simulink model "TRAS_nonlinear_controller"  (R2013a)
settings: Solver=ode5  SolverMode=SingleTasking  StartTime=0.0  StopTime=stop_time  FixedStep=sampling_time  RelTol=1e-3  AbsTol=1e-6
values from neighbouring files (symbols this model uses):
  A = 0.0552    [momentsOfInertia.m]
  B = 0.0599    [momentsOfInertia.m]
  C = 0.0084    [momentsOfInertia.m]
  D = (mmr + mms + mm / 3) * lm^2 + (mtr + mts + mt / 3) * lt^2    (= 0.0224143186667)    [momentsOfInertia.m]
  derivative_pole_tc = 10 * sampling_time    (= 0.1)    [TRAS_closed_loop.m]
  F = mms * rms^2 + mts * rts^2    (= 0.002355075)    [momentsOfInertia.m]
  Fh_force_grid = polyval(Fh, Fh_omega_grid)    [thrustForcesDependencies.m]
  Fh_omega_grid = linspace(-8000, 8000, 1e4)    [thrustForcesDependencies.m]
  Fv_force_grid = polyval(Fv, Fv_omega_grid)    [thrustForcesDependencies.m]
  Fv_omega_grid = linspace(-4000, 4000, 1e4)    [thrustForcesDependencies.m]
  g = 9.81    [TRAS_closed_loop.m]    (also in TRAS_controller.m; TRAS_process.m)
  Jv = D + E + F    (= 0.0253918936667)    [momentsOfInertia.m]
  kdh = 2 * zetah * wnh + poleh    (= 5.07276507277)    [TRAS_closed_loop.m]
  kdv = 2 * zetav * wnv + polev    (= 5.76397515528)    [TRAS_closed_loop.m]
  ki_inner = wn_inner^2    (= 19.7530864198)    [TRAS_closed_loop.m]
  kih = poleh * wnh^2    (= 2.0128563833)    [TRAS_closed_loop.m]
  kiv = polev * wnv^2    (= 3.43518684699)    [TRAS_closed_loop.m]
  kp_inner = 2 * zeta_inner * wn_inner    (= 8)    [TRAS_closed_loop.m]
  kph = wnh^2 + 2 * zetah * wnh * poleh    (= 6.9847554255)    [TRAS_closed_loop.m]
  kpv = wnv^2 + 2 * zetav * wnv * polev    (= 8.93792677752)    [TRAS_closed_loop.m]
  L = (mmr + mms + mm / 4) * lm^2 + (mtr + mts + mt / 4) * lt^2 - mcb * lcb^2 - mb / 4 * lb^2    (= 0.021593306)    [momentsOfInertia.m]
  lm = 0.202    [momentsOfInertia.m]
  lt = 0.216    [momentsOfInertia.m]
undefined symbols (not defined in the file): rtdac4pcibaseaddress
settings Model: SimulationMode=external  ExtModeTrigDuration=12000  ExtModeTrigLevel=0.400000  Creator=jims  LastModifiedBy=calc2
settings DataIOCC: ExternalInput=[]  InitialState=[]  LimitDataPoints=off  MaxDataPoints=5000  SignalLoggingSaveFormat=ModelDataLogs  SaveOutput=off  SaveTime=off  SignalLoggingName=sigsOut
settings OptimizationCC: BooleanDataType=off  ExpressionDepthLimit=2147483647  InitFltsAndDblsToZero=on
settings DebuggingCC: SaveWithParameterizedLinksMsg=none  MergeDetectMultiDrivingBlocksExec=error  SolverPrmCheckMsg=none  MultiTaskDSMMsg=warning  MultiTaskCondExecSysMsg=none  IntegerOverflowMsg=none  FcnCallInpInsideContextMsg=EnableAllAsWarning  StrictBusMsg=None
settings HardwareCC: TargetEndianess=LittleEndian  TargetHWDeviceType=MATLAB Host
settings RTWCC: SystemTargetFile=rtwin.tlc  TemplateMakefile=rtwin.tmf  Description=Real-Time Windows Target  ProcessScript=rtwin_make_rtw_hook  IncludeERTFirstTime=on
settings RTWinTargetCC: TargetFcnLib=ansi_tfl_tmw.mat  TargetLibSuffix=_rtwin.lib  TargetPreCompLibLocation=C:\Program Files\MATLAB\R2013a\toolbox\rtw\targets\rtwin\lib\win32  CodeReplacementLibrary=ANSI_C  ModelReferenceCompliant=off  CompOptLevelCompliant=off  RTWinDir=C:/PROGRA~1/MATLAB/R2013a/toolbox/rtw/targets/rtwin  TargetArch=win32

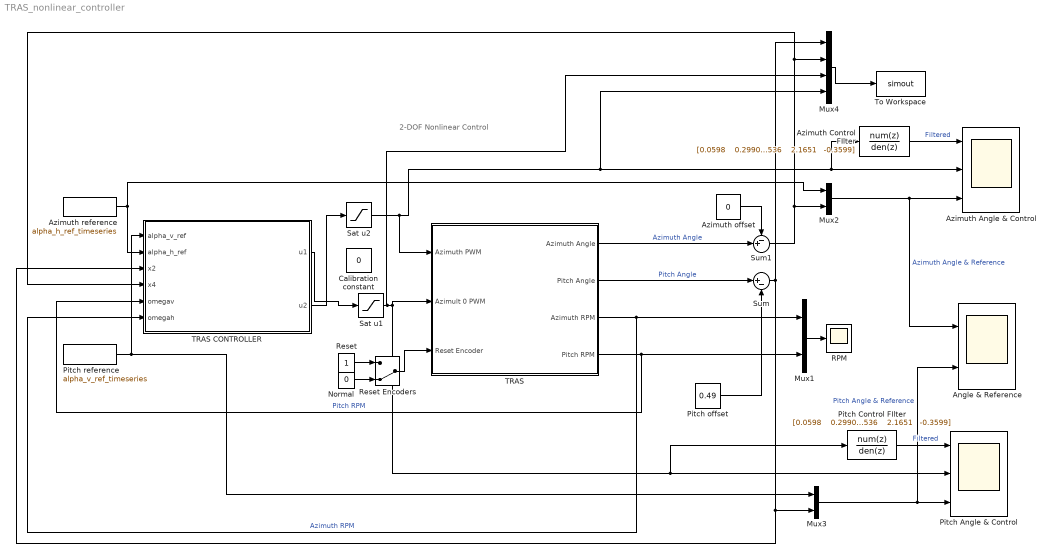
== system TRAS_nonlinear_controller ==
  note: 2-DOF Nonlinear Control
  Angle & Reference : Scope  NumInputPorts=2
      settings: TimeRange=60  YMin=-0.6~-0.55  YMax=0.8~0.55  SaveName=AngleReference_  MaxDataPoints=12000
  Azimuth Angle & Control : Scope  NumInputPorts=3
      settings: TimeRange=90  YMin=-0.4~-0.5~-1  YMax=-0.225~0.5~1  SaveName=AngleCtrl_  MaxDataPoints=12000
  Azimuth Control FIlter : DiscreteTransferFcn  Numerator="[0.0598    0.2990    0.5980    0.5980    0.2990    0.0598] * 1e-3"  Denominator="[1.0000   -3.9845    6.4349   -5.2536    2.1651   -0.3599]"  SampleTime=0.01
  Azimuth offset : Constant  Value=0
  "Azimuth reference " : FromWorkspace  VariableName=alpha_h_ref_timeseries  SampleTime=0
  Calibration constant : Constant  Value=0
  Mux1 : Mux  Inputs=2
  Mux2 : Mux  Inputs=2
  Mux3 : Mux  Inputs=2
  Mux4 : Mux
  Normal : Constant  Value=0
  Pitch Angle & Control : Scope  NumInputPorts=3
      settings: TimeRange=90  YMin=2.77556e-17~-0.1~-0.5  YMax=0.75~0.9~0.35  SaveName=AngleCtrl1_  MaxDataPoints=12000
  Pitch Control FIlter : DiscreteTransferFcn  Numerator="[0.0598    0.2990    0.5980    0.5980    0.2990    0.0598] * 1e-3"  Denominator="[1.0000   -3.9845    6.4349   -5.2536    2.1651   -0.3599]"  SampleTime=0.01
  Pitch offset : Constant  Value=0.49
  Pitch reference : FromWorkspace  VariableName=alpha_v_ref_timeseries  SampleTime=0
  RPM : Scope
      settings: TimeRange=90  YMin=-6000  YMax=7000  SaveName=RPM_  MaxDataPoints=12000
  Reset : Constant
  Reset Encoders : ManualSwitch  CurrentSetting=0
  Sat u1 : Saturate  UpperLimit=1  LowerLimit=-1
  Sat u2 : Saturate  UpperLimit=1  LowerLimit=-1
  Sum : Sum  Inputs=|+-
  Sum1 : Sum  Inputs=-+|
  TRAS : Subsystem  mask{BaseAddress=rtdac4pcibaseaddress, T0=0.01}
      mask prompts: BaseAddress "Base Address:"; T0 "Sampling Period:"
      mask Display: image(imread('TRAS.JPG'))
  TRAS CONTROLLER : Subsystem
  To Workspace : ToWorkspace  VariableName=simout  SampleTime=-1  SaveFormat=Structure With Time
  wires:
  Pitch Control FIlter/1 -> Pitch Angle & Control/1  "Filtered"
  Mux3/1 -> Pitch Angle & Control/3, Angle & Reference/2  "Pitch Angle & Reference"
  Mux1/1 -> RPM/1
  Sat u2/1 -> TRAS/1(Azimuth PWM), Mux4/4, Azimuth Angle & Control/2, Azimuth Control FIlter/1
  Sat u1/1 -> Mux4/3, TRAS/2(Azimult 0 PWM), Pitch Angle & Control/2, Pitch Control FIlter/1
  Azimuth Control FIlter/1 -> Azimuth Angle & Control/1  "Filtered"
  Mux2/1 -> Azimuth Angle & Control/3, Angle & Reference/1  "Azimuth Angle & Reference"
  Reset Encoders/1 -> TRAS/3(Reset Encoder)
  Reset/1 -> Reset Encoders/1
  Normal/1 -> Reset Encoders/2
  TRAS/4(Pitch RPM) -> TRAS CONTROLLER/5(omegav), Mux1/2  "Pitch RPM"
  TRAS/3(Azimuth RPM) -> TRAS CONTROLLER/6(omegah), Mux1/1  "Azimuth RPM"
  "Azimuth reference "/1 -> TRAS CONTROLLER/2(alpha_h_ref), Mux2/1
  Pitch reference/1 -> TRAS CONTROLLER/1(alpha_v_ref), Mux3/1
  Sum/1 -> TRAS CONTROLLER/3(x2), Mux3/2, Mux4/1
  Pitch offset/1 -> Sum/2
  Mux4/1 -> To Workspace/1
  Azimuth offset/1 -> Sum1/1
  Sum1/1 -> Mux4/2, TRAS CONTROLLER/4(x4), Mux2/2
  TRAS CONTROLLER/2(u2) -> Sat u2/1
  TRAS CONTROLLER/1(u1) -> Sat u1/1
  TRAS/1(Azimuth Angle) -> Sum1/2  "Azimuth Angle"
  TRAS/2(Pitch Angle) -> Sum/1  "Pitch Angle"

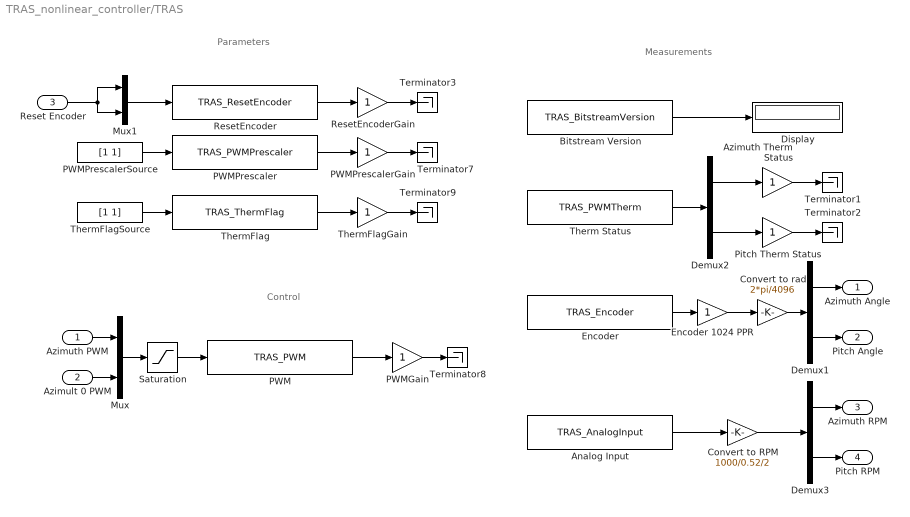
== system TRAS_nonlinear_controller/TRAS ==
  note: Parameters
  note: Control
  note: Measurements
  Azimuth PWM : Inport
  Azimult 0 PWM : Inport  Port=2
  Reset Encoder : Inport  Port=3
  Analog Input : S-Function  FunctionName=TRAS_AnalogInput  Parameters=BaseAddress, [1 0], [1 1], T0  EnableBusSupport=off
  Azimuth Therm Status : Gain  SaturateOnIntegerOverflow=on  OutDataTypeStr=Inherit: Same as input  ParamDataTypeStr=Inherit: Same as input
  Bitstream Version : S-Function  FunctionName=TRAS_BitstreamVersion  Parameters=BaseAddress, T0  EnableBusSupport=off
  Convert to RPM : Gain  Gain=1000/0.52/2  SaturateOnIntegerOverflow=on  OutDataTypeStr=Inherit: Same as input  ParamDataTypeStr=Inherit: Same as input
  Convert to rad : Gain  Gain=2*pi/4096  SaturateOnIntegerOverflow=on  OutDataTypeStr=Inherit: Same as input  ParamDataTypeStr=Inherit: Same as input
  Demux1 : Demux  Outputs=2
  Demux2 : Demux  Outputs=2
  Demux3 : Demux  Outputs=2
  Display : Display
  Encoder : S-Function  FunctionName=TRAS_Encoder  Parameters=BaseAddress, T0  EnableBusSupport=off
  Encoder 1024 PPR : Gain  SaturateOnIntegerOverflow=on  OutDataTypeStr=Inherit: Same as input  ParamDataTypeStr=Inherit: Same as input
  Mux : Mux  Inputs=2
  Mux1 : Mux  Inputs=2
  PWM : S-Function  FunctionName=TRAS_PWM  Parameters=BaseAddress, T0  EnableBusSupport=off
  PWMGain : Gain  SaturateOnIntegerOverflow=on  OutDataTypeStr=Inherit: Same as input  ParamDataTypeStr=Inherit: Same as input
  PWMPrescaler : S-Function  FunctionName=TRAS_PWMPrescaler  Parameters=BaseAddress, T0  EnableBusSupport=off
  PWMPrescalerGain : Gain  SaturateOnIntegerOverflow=on  OutDataTypeStr=Inherit: Same as input  ParamDataTypeStr=Inherit: Same as input
  PWMPrescalerSource : Constant  Value=[1 1]
  Pitch Therm Status : Gain  SaturateOnIntegerOverflow=on  OutDataTypeStr=Inherit: Same as input  ParamDataTypeStr=Inherit: Same as input
  ResetEncoder : S-Function  FunctionName=TRAS_ResetEncoder  Parameters=BaseAddress, T0  EnableBusSupport=off
  ResetEncoderGain : Gain  SaturateOnIntegerOverflow=on  OutDataTypeStr=Inherit: Same as input  ParamDataTypeStr=Inherit: Same as input
  Saturation : Saturate  UpperLimit=1  LowerLimit=-1
  Terminator{1..3,7..9} (6 alike) : Terminator
  Therm Status : S-Function  FunctionName=TRAS_PWMTherm  Parameters=BaseAddress, T0  EnableBusSupport=off
  "ThermFlag " : S-Function  FunctionName=TRAS_ThermFlag  Parameters=BaseAddress, T0  EnableBusSupport=off
  ThermFlagGain : Gain  SaturateOnIntegerOverflow=on  OutDataTypeStr=Inherit: Same as input  ParamDataTypeStr=Inherit: Same as input
  ThermFlagSource : Constant  Value=[1 1]
  Azimuth Angle : Outport  InitialOutput=0
  Pitch Angle : Outport  Port=2  InitialOutput=0
  Azimuth RPM : Outport  Port=3  InitialOutput=0
  Pitch RPM : Outport  Port=4  InitialOutput=0
  wires:
  Encoder 1024 PPR/1 -> Convert to rad/1
  Encoder/1 -> Encoder 1024 PPR/1
  Saturation/1 -> PWM/1
  Mux/1 -> Saturation/1
  PWM/1 -> PWMGain/1
  PWMGain/1 -> Terminator8/1
  ResetEncoder/1 -> ResetEncoderGain/1
  PWMPrescaler/1 -> PWMPrescalerGain/1
  Mux1/1 -> ResetEncoder/1
  PWMPrescalerSource/1 -> PWMPrescaler/1
  ResetEncoderGain/1 -> Terminator3/1
  PWMPrescalerGain/1 -> Terminator7/1
  Azimult 0 PWM/1 -> Mux/2
  Azimuth PWM/1 -> Mux/1
  Demux1/2 -> Pitch Angle/1
  Convert to rad/1 -> Demux1/1
  Demux1/1 -> Azimuth Angle/1
  Therm Status/1 -> Demux2/1
  Demux2/2 -> Pitch Therm Status/1
  Demux2/1 -> Azimuth Therm Status/1
  Azimuth Therm Status/1 -> Terminator1/1
  Pitch Therm Status/1 -> Terminator2/1
  Bitstream Version/1 -> Display/1
  Analog Input/1 -> Convert to RPM/1
  Demux3/2 -> Pitch RPM/1
  Demux3/1 -> Azimuth RPM/1
  Reset Encoder/1 -> Mux1/1, Mux1/2
  Convert to RPM/1 -> Demux3/1
  "ThermFlag "/1 -> ThermFlagGain/1
  ThermFlagSource/1 -> "ThermFlag "/1
  ThermFlagGain/1 -> Terminator9/1

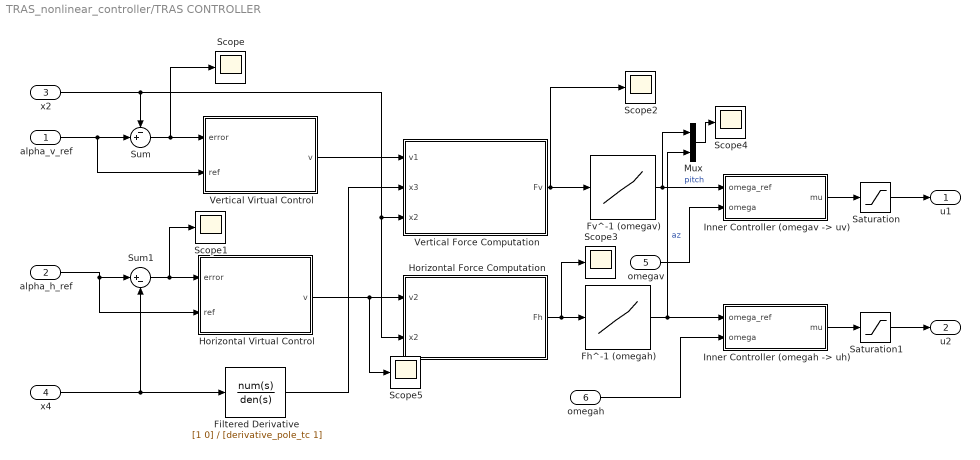
== system TRAS_nonlinear_controller/TRAS CONTROLLER ==
  alpha_v_ref : Inport
  alpha_h_ref : Inport  Port=2
  x2 : Inport  Port=3
  x4 : Inport  Port=4
  omegav : Inport  Port=5
  omegah : Inport  Port=6
  Fh^-1 (omegah) : Lookup_n-D  NumberOfTableDimensions=1  BreakpointsForDimension1=Fh_force_grid  Table=Fh_omega_grid  ExtrapMethod=Clip  RndMeth=Simplest  InputSameDT=on
  Filtered Derivative : TransferFcn  Numerator=[1 0]  Denominator=[derivative_pole_tc 1]
  Fv^-1 (omegav) : Lookup_n-D  NumberOfTableDimensions=1  BreakpointsForDimension1=Fv_force_grid  Table=Fv_omega_grid  ExtrapMethod=Clip  RndMeth=Simplest  InputSameDT=on
  Horizontal Force Computation : MATLAB Function  TreatAsAtomicUnit=on
  Horizontal Virtual Control : Subsystem
  "Inner Controller (omegah -> uh)" : Subsystem
  "Inner Controller (omegav -> uv)" : Subsystem
  Mux : Mux  Inputs=2
  Saturation : Saturate  UpperLimit=0.98  LowerLimit=-0.98
  Saturation1 : Saturate  UpperLimit=0.98  LowerLimit=-0.98
  Scope{,1..5} (6 alike) : Scope
      Scope1 settings: SaveName=ScopeData2
      Scope2 settings: SaveName=ScopeData4
      Scope3 settings: SaveName=ScopeData5
      Scope4 settings: ShowLegends=on  SaveName=ScopeData7
      Scope5 settings: SaveName=ScopeData8
  Sum : Sum  Inputs=-+|
  Sum1 : Sum  Inputs=|+-
  Vertical Force Computation : MATLAB Function  TreatAsAtomicUnit=on
  Vertical Virtual Control : Subsystem
  u1 : Outport
  u2 : Outport  Port=2
  wires:
  Filtered Derivative/1 -> Vertical Force Computation/2(x3)
  Vertical Virtual Control/1(v) -> Vertical Force Computation/1(v1)
  x2/1 -> Horizontal Force Computation/2(x2), Vertical Force Computation/3(x2), Sum/1
  Horizontal Virtual Control/1(v) -> Scope5/1, Horizontal Force Computation/1(v2)
  x4/1 -> Sum1/2, Filtered Derivative/1
  alpha_v_ref/1 -> Vertical Virtual Control/2(ref), Sum/2
  alpha_h_ref/1 -> Horizontal Virtual Control/2(ref), Sum1/1
  Sum1/1 -> Horizontal Virtual Control/1(error), Scope1/1
  "Inner Controller (omegav -> uv)"/1(mu) -> Saturation/1
  "Inner Controller (omegah -> uh)"/1(mu) -> Saturation1/1
  Sum/1 -> Scope/1, Vertical Virtual Control/1(error)
  Horizontal Force Computation/1(Fh) -> Scope3/1, Fh^-1 (omegah)/1
  Fv^-1 (omegav)/1 -> "Inner Controller (omegav -> uv)"/1(omega_ref), Mux/1  "pitch"
  Fh^-1 (omegah)/1 -> "Inner Controller (omegah -> uh)"/1(omega_ref), Mux/2  "az"
  Saturation/1 -> u1/1
  Saturation1/1 -> u2/1
  Mux/1 -> Scope4/1
  omegav/1 -> "Inner Controller (omegav -> uv)"/2(omega)
  omegah/1 -> "Inner Controller (omegah -> uh)"/2(omega)
  Vertical Force Computation/1(Fv) -> Fv^-1 (omegav)/1, Scope2/1

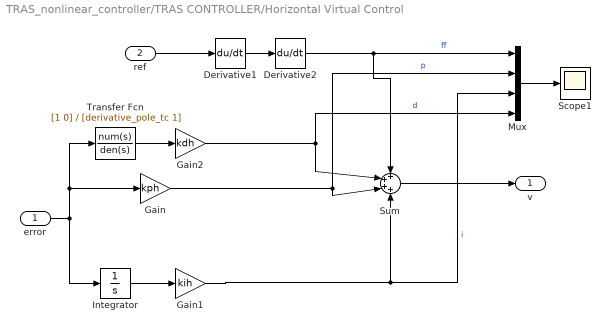
== system TRAS_nonlinear_controller/TRAS CONTROLLER/Horizontal Virtual Control ==
  error : Inport
  ref : Inport  Port=2
  Derivative1 : Derivative
  Derivative2 : Derivative
  Gain : Gain  Gain=kph
  Gain1 : Gain  Gain=kih
  Gain2 : Gain  Gain=kdh
  Integrator : Integrator  UpperSaturationLimit=0.2  LowerSaturationLimit=-0.2
  Mux : Mux
  Scope1 : Scope
      settings: ShowLegends=on  YMin=-0.2  YMax=0.175  SaveName=ScopeData10
  Sum : Sum  Inputs=++++
  Transfer Fcn : TransferFcn  Numerator=[1 0]  Denominator=[derivative_pole_tc 1]
  v : Outport
  wires:
  Integrator/1 -> Gain1/1
  ref/1 -> Derivative1/1
  Derivative1/1 -> Derivative2/1
  error/1 -> Integrator/1, Gain/1, Transfer Fcn/1
  Transfer Fcn/1 -> Gain2/1
  Derivative2/1 -> Sum/1, Mux/1  "ff"
  Sum/1 -> v/1
  Mux/1 -> Scope1/1
  Gain2/1 -> Mux/4, Sum/2  "d"
  Gain/1 -> Sum/3, Mux/2  "p"
  Gain1/1 -> Mux/3, Sum/4  "i"

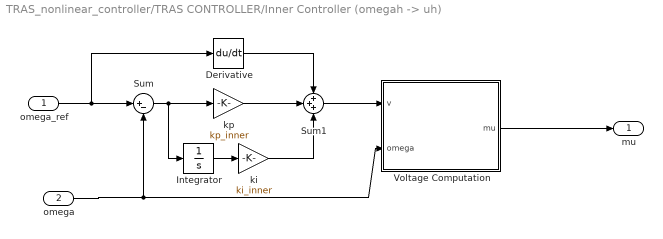
== system TRAS_nonlinear_controller/TRAS CONTROLLER/Inner Controller (omegah -> uh) ==
  omega_ref : Inport
  omega : Inport  Port=2
  Derivative : Derivative
  Integrator : Integrator
  Sum : Sum  Inputs=|+-
  Sum1 : Sum  Inputs=+++
  Voltage Computation : MATLAB Function  TreatAsAtomicUnit=on
  ki : Gain  Gain=ki_inner
  kp : Gain  Gain=kp_inner
  mu : Outport
  wires:
  ki/1 -> Sum1/3
  Integrator/1 -> ki/1
  Voltage Computation/1(mu) -> mu/1
  Sum1/1 -> Voltage Computation/1(v)
  Derivative/1 -> Sum1/1
  kp/1 -> Sum1/2
  Sum/1 -> kp/1, Integrator/1
  omega_ref/1 -> Sum/1, Derivative/1
  omega/1 -> Voltage Computation/2(omega), Sum/2

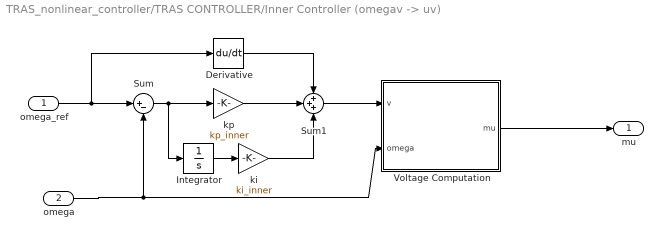
== system TRAS_nonlinear_controller/TRAS CONTROLLER/Inner Controller (omegav -> uv) ==
  omega_ref : Inport
  omega : Inport  Port=2
  Derivative : Derivative
  Integrator : Integrator
  Sum : Sum  Inputs=|+-
  Sum1 : Sum  Inputs=+++
  Voltage Computation : MATLAB Function  TreatAsAtomicUnit=on
  ki : Gain  Gain=ki_inner
  kp : Gain  Gain=kp_inner
  mu : Outport
  wires:
  omega/1 -> Sum/2, Voltage Computation/2(omega)
  omega_ref/1 -> Derivative/1, Sum/1
  Sum/1 -> Integrator/1, kp/1
  kp/1 -> Sum1/2
  Derivative/1 -> Sum1/1
  Sum1/1 -> Voltage Computation/1(v)
  Voltage Computation/1(mu) -> mu/1
  Integrator/1 -> ki/1
  ki/1 -> Sum1/3

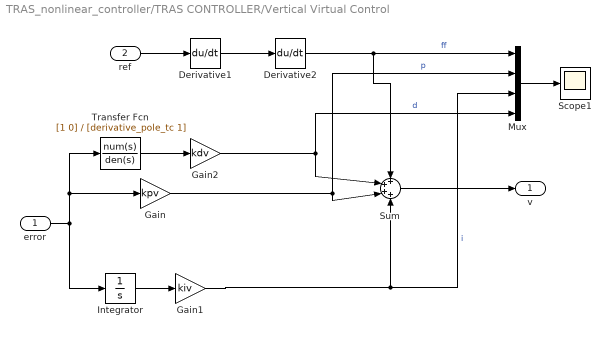
== system TRAS_nonlinear_controller/TRAS CONTROLLER/Vertical Virtual Control ==
  error : Inport
  ref : Inport  Port=2
  Derivative1 : Derivative
  Derivative2 : Derivative
  Gain : Gain  Gain=kpv
  Gain1 : Gain  Gain=kiv
  Gain2 : Gain  Gain=kdv
  Integrator : Integrator  UpperSaturationLimit=0.2  LowerSaturationLimit=-0.2
  Mux : Mux
  Scope1 : Scope
      settings: ShowLegends=on  YMin=-0.2  YMax=0.175  SaveName=ScopeData6
  Sum : Sum  Inputs=++++
  Transfer Fcn : TransferFcn  Numerator=[1 0]  Denominator=[derivative_pole_tc 1]
  v : Outport
  wires:
  Integrator/1 -> Gain1/1
  ref/1 -> Derivative1/1
  Derivative1/1 -> Derivative2/1
  error/1 -> Integrator/1, Gain/1, Transfer Fcn/1
  Transfer Fcn/1 -> Gain2/1
  Derivative2/1 -> Sum/1, Mux/1  "ff"
  Sum/1 -> v/1
  Mux/1 -> Scope1/1
  Gain2/1 -> Mux/4, Sum/2  "d"
  Gain/1 -> Sum/3, Mux/2  "p"
  Gain1/1 -> Mux/3, Sum/4  "i"

== matlab function TRAS_nonlinear_controller/TRAS CONTROLLER/Vertical Force Computation ==
  data: Fv output; v1 input; x3 input; x2 input; Jv parameter; L parameter; g parameter; A parameter; B parameter; C parameter; lm parameter
function Fv = verticalForceComputation(v1, x3, x2, Jv, L, g, A, B, C, lm)

Fv = 1 / lm * (v1 * Jv + x3^2 / 2 * L * sin(2 * x2) - g * ((A-B)*cos(x2) - C*sin(x2)));

== matlab function TRAS_nonlinear_controller/TRAS CONTROLLER/Horizontal Force Computation ==
  data: v2 input; Fh output; x2 input; lt parameter; D parameter; E parameter; F parameter
function Fh = horizontalForceComputation(v2, x2, lt, D, E, F)

Fh = v2 / (lt * cos(x2)) * (D * cos(x2)^2 + E * sin(x2)^2 + F);

== matlab function TRAS_nonlinear_controller/TRAS CONTROLLER/Inner Controller (omegav -> uv)/Voltage Computation ==
  data: v input; mu output; omega input; Thetav parameter
function mu = PWMComputation(v, omega, Thetav)

%case1 : suppose mu >= 0
mu = (v + Thetav(3) * omega + omega * abs(omega) * Thetav(4)) / (Thetav(1) - Thetav(2));

if(mu < 0) %case 2: mu < 0
    mu = (v + Thetav(3) * omega + omega * abs(omega) * Thetav(4)) / (Thetav(1) + Thetav(2));
end

== matlab function TRAS_nonlinear_controller/TRAS CONTROLLER/Inner Controller (omegah -> uh)/Voltage Computation ==
  data: v input; mu output; omega input; Thetah parameter
function mu = PWMComputation(v, omega, Thetah)

%case1 : suppose mu >= 0
mu = (v + Thetah(3) * omega + omega * abs(omega) * Thetah(4)) / (Thetah(1) - Thetah(2));

if(mu < 0) %case 2: mu < 0
    mu = (v + Thetah(3) * omega + omega * abs(omega) * Thetah(4)) / (Thetah(1) + Thetah(2));
end
